simulink model "exp3_3_PID"  (R2020b)
settings: Solver=ode3  StartTime=0.0  StopTime=12  FixedStep=0.001  RelTol=1e-3
undefined symbols (not defined in the file): DiscIntNeverNeededParam, drv, enable_anti_windup, Kd, Ki, Kp, Kw, National_Instruments, PCI, sens, step_height, step_time, Tl, Ts
libraries: simulink x3, sldrtlib x3
settings Model: SimulationMode=external  ExtModeTrigDuration=150000  Creator=controlsystemsuser  LastModifiedBy=grandinmat
settings DataIOCC: ReturnWorkspaceOutputs=off
settings RTWCC: Description=Simulink Desktop Real-Time  SystemTargetFile=sldrt.tlc  TemplateMakefile=sldrt.tmf  RTWCompilerOptimization=on
settings CodeAppCC: MaxIdLength=95
settings SimulinkDesktopRealTimeCC: TargetPreCompLibLocation=C:\Program Files\MATLAB\R2020b\toolbox\sldrt\lib\win64

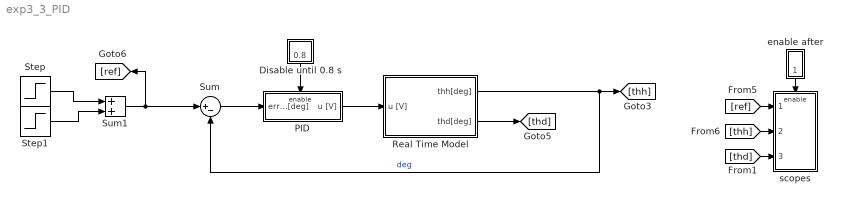
== system exp3_3_PID ==
  Disable until 0.8 s : Subsystem
  PID : Subsystem
  Real Time Model : Subsystem
  Step : Step  Time=step_time  After=step_height  SampleTime=0
  Step1 : Step  Time=step_time+5  After=-step_height  SampleTime=0
  Sum : Sum  Inputs=|+-
  Sum1 : Sum
  enable after : Subsystem
  scopes : Subsystem
  wires:
  enable after/1(1.0 s) -> scopes/Enable
  [thd] -> scopes/3(thd[deg])
  [thh] -> scopes/2(thh[deg])
  [ref] -> scopes/1(ref[deg])
  Step1/1 -> Sum1/2
  Step/1 -> Sum1/1
  Sum1/1 -> Sum/1, [ref]
  Sum/1 -> PID/1(error [deg])
  Disable until 0.8 s/1(0.8) -> PID/Enable
  PID/1(u [V]) -> Real Time Model/1(u [V])
  Real Time Model/2(thd[deg]) -> [thd]
  Real Time Model/1(thh[deg]) -> [thh], Sum/2  "deg"

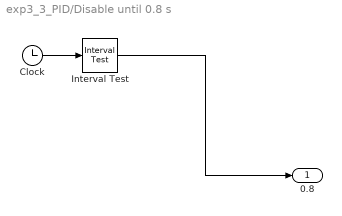
== system exp3_3_PID/Disable until 0.8 s ==
  Clock : Clock
  Interval Test : simulink/Logic and Bit Operations/Interval Test  IntervalClosedRight=on  uplimit=inf  IntervalClosedLeft=on  lowlimit=0.8  OutDataTypeStr=boolean
  0.8 : Outport
  wires:
  Interval Test/1 -> 0.8/1
  Clock/1 -> Interval Test/1

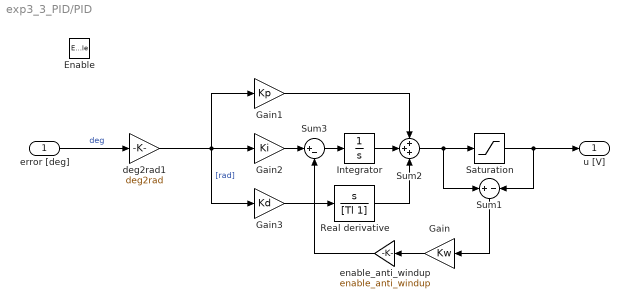
== system exp3_3_PID/PID ==
  error [deg] : Inport
  Enable : EnablePort
  Gain : Gain  Gain=Kw
  Gain1 : Gain  Gain=Kp
  Gain2 : Gain  Gain=Ki
  Gain3 : Gain  Gain=Kd
  Integrator : Integrator
  Real derivative : TransferFcn  Numerator=[1 0]  Denominator=[Tl 1]
  Saturation : Saturate  UpperLimit=drv.outmax  LowerLimit=-drv.outmax  LinearizeAsGain=off
  Sum1 : Sum  Inputs=+|-
  Sum2 : Sum  Inputs=+++
  Sum3 : Sum  Inputs=|+-
  deg2rad1 : Gain  Gain=deg2rad
  enable_anti_windup : Gain  Gain=enable_anti_windup
  u [V] : Outport
  wires:
  enable_anti_windup/1 -> Sum3/2
  Gain/1 -> enable_anti_windup/1
  Integrator/1 -> Sum2/2
  Sum3/1 -> Integrator/1
  Gain3/1 -> Real derivative/1
  Real derivative/1 -> Sum2/3
  Sum2/1 -> Saturation/1, Sum1/1
  Saturation/1 -> Sum1/2, u [V]/1
  Sum1/1 -> Gain/1
  Gain2/1 -> Sum3/1
  error [deg]/1 -> deg2rad1/1  "deg"
  Gain1/1 -> Sum2/1
  deg2rad1/1 -> Gain2/1, Gain1/1, Gain3/1  "[rad]"

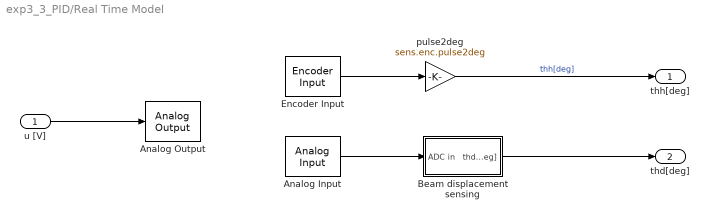
== system exp3_3_PID/Real Time Model ==
  u [V] : Inport
  Analog Input : sldrtlib/Analog Input  SampleTime=0.001  MaxMissedTicks=10  ShowMissedTicks=off  YieldWhenWaiting=off  DrvName=National_Instruments/PCI-6221  DrvAddress=4294967295  DrvOptions=[0 0 0 2 0]  Channels=[3,4]  RangeMode=1  VoltRange=2  DataType=1
      settings: AttributesFormatString=National Instruments\nPCI-6221 [auto]
  Analog Output : sldrtlib/Analog Output  SampleTime=0.001  MaxMissedTicks=10  ShowMissedTicks=off  YieldWhenWaiting=off  DrvName=National_Instruments/PCI-6221  DrvAddress=4294967295  DrvOptions=[0 0 0 2 0]  Channels=1  RangeMode=1  VoltRange=1  InitialValue=0  FinalValue=0
      settings: AttributesFormatString=National Instruments\nPCI-6221 [auto]
  Beam displacement sensing : Subsystem
  Encoder Input : sldrtlib/Encoder Input  SampleTime=0.001  MaxMissedTicks=10  ShowMissedTicks=off  YieldWhenWaiting=off  DrvName=National_Instruments/PCI-6221  DrvAddress=4294967295  DrvOptions=[0 0 0 2 0]  Channels=1  QuadMode=3  IndexPulse=1  InputFilter=Inf  DataType=1
      settings: AttributesFormatString=National Instruments\nPCI-6221 [auto]
  pulse2deg : Gain  Gain=sens.enc.pulse2deg
  thh[deg] : Outport
  thd[deg] : Outport  Port=2
  wires:
  Encoder Input/1 -> pulse2deg/1
  Beam displacement sensing/1(thd[deg]) -> thd[deg]/1
  Analog Input/1 -> Beam displacement sensing/1(ADC in)
  pulse2deg/1 -> thh[deg]/1  "thh[deg]"
  u [V]/1 -> Analog Output/1

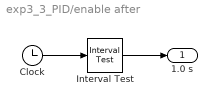
== system exp3_3_PID/enable after ==
  Clock : Clock
  Interval Test : simulink/Logic and Bit Operations/Interval Test  IntervalClosedRight=on  uplimit=inf  IntervalClosedLeft=on  lowlimit=1  OutDataTypeStr=boolean
  1.0 s : Outport
  wires:
  Interval Test/1 -> 1.0 s/1
  Clock/1 -> Interval Test/1

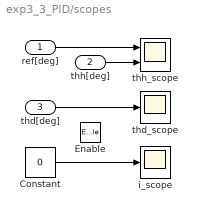
== system exp3_3_PID/scopes ==
  ref[deg] : Inport
  thh[deg] : Inport  Port=2
  thd[deg] : Inport  Port=3
  Enable : EnablePort
  Constant : Constant  Value=0
  i_scope : Scope
  thd_scope : Scope
  thh_scope : Scope  NumInputPorts=2
  wires:
  thd[deg]/1 -> thd_scope/1
  Constant/1 -> i_scope/1
  thh[deg]/1 -> thh_scope/2
  ref[deg]/1 -> thh_scope/1

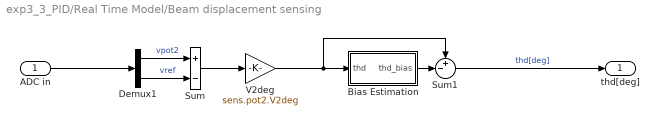
== system exp3_3_PID/Real Time Model/Beam displacement sensing ==
  ADC in : Inport
  Bias Estimation : Subsystem
  Demux1 : Demux  Outputs=2
  Sum : Sum  Inputs=+-
  Sum1 : Sum  Inputs=+-|
  V2deg : Gain  Gain=sens.pot2.V2deg
  thd[deg] : Outport
  wires:
  Bias Estimation/1(thd_bias) -> Sum1/2
  Sum/1 -> V2deg/1
  Demux1/1 -> Sum/1  "vpot2"
  Demux1/2 -> Sum/2  "vref"
  Sum1/1 -> thd[deg]/1  "thd[deg]"
  V2deg/1 -> Sum1/1, Bias Estimation/1(thd)
  ADC in/1 -> Demux1/1

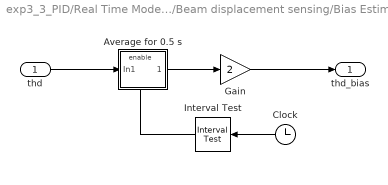
== system exp3_3_PID/Real Time Model/Beam displacement sensing/Bias Estimation ==
  thd : Inport
  Average for 0.5 s : Subsystem
  Clock : Clock
  Gain : Gain  Gain=2
  Interval Test : simulink/Logic and Bit Operations/Interval Test  IntervalClosedRight=on  uplimit=0.7  IntervalClosedLeft=on  lowlimit=0.2  OutDataTypeStr=boolean
  thd_bias : Outport
  wires:
  Interval Test/1 -> Average for 0.5 s/Enable
  thd/1 -> Average for 0.5 s/1(In1)
  Clock/1 -> Interval Test/1
  Average for 0.5 s/1(Out1) -> Gain/1
  Gain/1 -> thd_bias/1

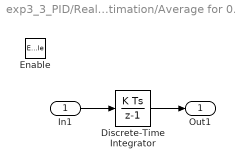
== system exp3_3_PID/Real Time Model/Beam displacement sensing/Bias Estimation/Average for 0.5 s ==
  In1 : Inport
  Enable : EnablePort
  Discrete-Time Integrator : DiscreteIntegrator  SampleTime=Ts  ICPrevOutput=DiscIntNeverNeededParam  ICPrevScaledInput=DiscIntNeverNeededParam
  Out1 : Outport
  wires:
  In1/1 -> Discrete-Time Integrator/1
  Discrete-Time Integrator/1 -> Out1/1
